simulink model "modified_bouc_wen_sdof"  (R2020a)
settings: Solver=VariableStepAuto  StartTime=0.0  StopTime=10.0  RelTol=1e-3
values from neighbouring files (symbols this model uses):
  A = 301    [modified_bouc_wen_model_parameters.m]
  alpha_a = 140    [modified_bouc_wen_model_parameters.m]
  alpha_b = 695    [modified_bouc_wen_model_parameters.m]
  beta1 = 363    [modified_bouc_wen_model_parameters.m]
  c_0a = 21    [modified_bouc_wen_model_parameters.m]
  c_0b = 3.5    [modified_bouc_wen_model_parameters.m]
  c_1a = 283    [modified_bouc_wen_model_parameters.m]
  c_1b = 2.95    [modified_bouc_wen_model_parameters.m]
  C_s = dr*2*sqrt(m_s*K_s)    [modified_bouc_wen_model_parameters.m]
  eta1 = 190    [modified_bouc_wen_model_parameters.m]
  gamma1 = 363    [modified_bouc_wen_model_parameters.m]
  k0 = 46.9    [modified_bouc_wen_model_parameters.m]
  k1 = 80000    [PID_controller_tov.m]    (also in modified_bouc_wen_model_parameters.m = 5)
  K_s = m_s*((2*pi/T)^2)    (= 155.22913802)    [modified_bouc_wen_model_parameters.m]
  m_s = 98.3    [modified_bouc_wen_model_parameters.m]
  n = 2    [modified_bouc_wen_model_parameters.m]
  x0 = 14.3    [modified_bouc_wen_model_parameters.m]
settings Model: Creator=siddh  LastModifiedBy=siddh

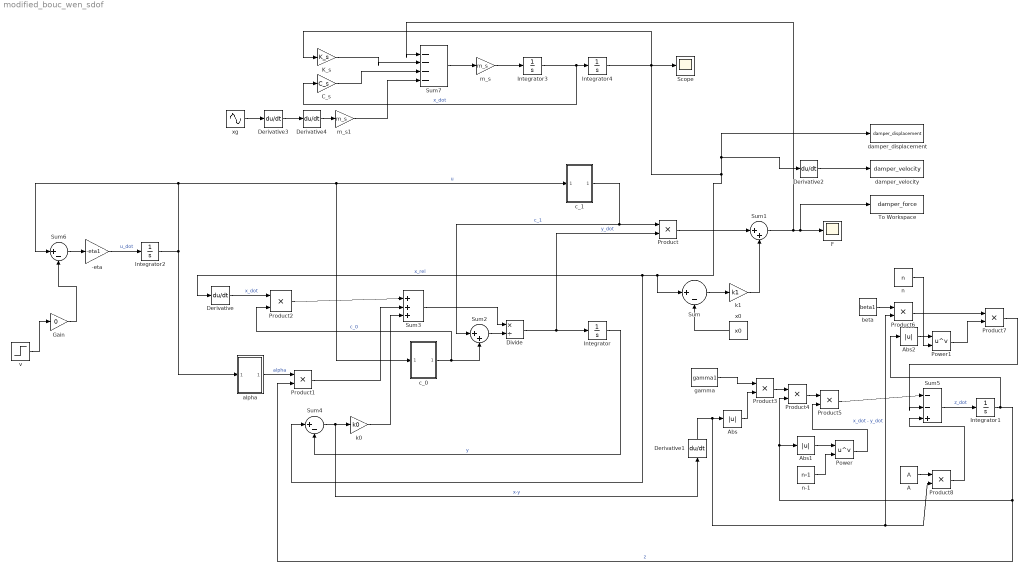
== system modified_bouc_wen_sdof ==
  -eta : Gain  Gain=-eta1
  A : Constant  Value=A
  Abs : Abs
  Abs1 : Abs
  Abs2 : Abs
  C_s : Gain  Gain=C_s
  Derivative{,1..4} (5 alike) : Derivative
  Divide : Product  Inputs=*/
  F : Scope
  Gain : Gain  Gain=0
  Integrator{,1..4} (5 alike) : Integrator
  K_s : Gain  Gain=K_s
  Power : Math  Operator=pow  SaturateOnIntegerOverflow=on
  Power1 : Math  Operator=pow  SaturateOnIntegerOverflow=on
  Product{,1..8} (9 alike) : Product
  Scope : Scope
  Sum : Sum  Inputs=|+-
  Sum1 : Sum  Inputs=|++
  Sum2 : Sum  Inputs=|++
  Sum3 : Sum  Inputs=|+++
  Sum4 : Sum  Inputs=|+-
  Sum5 : Sum  Inputs=|--+
  Sum6 : Sum  Inputs=|+-
  Sum7 : Sum  Inputs=|----
  To Workspace : ToWorkspace  VariableName=damper_force  SampleTime=-1
  alpha : Subsystem
  beta : Constant  Value=beta1
  c_0 : Subsystem
  c_1 : Subsystem
  damper_displacement : ToWorkspace  VariableName=damper_displacement  SampleTime=-1
  damper_velocity : ToWorkspace  VariableName=damper_velocity  SampleTime=-1
  gamma : Constant  Value=gamma1
  k0 : Gain  Gain=k0
  k1 : Gain  Gain=k1
  m_s : Gain  Gain=m_s
  m_s1 : Gain  Gain=m_s
  n : Constant  Value=n
  n-1 : Constant  Value=n-1
  v : Step  SampleTime=0
  x0 : Constant  Value=x0
  xg : Sin  Amplitude=0.75  Frequency=2*pi*4  SampleTime=0
  wires:
  m_s/1 -> Integrator3/1
  Product8/1 -> Sum5/3
  m_s1/1 -> Sum7/4
  Derivative4/1 -> m_s1/1
  A/1 -> Product8/1
  xg/1 -> Derivative3/1
  Product5/1 -> Sum5/1
  Product4/1 -> Product5/1
  C_s/1 -> Sum7/3
  K_s/1 -> Sum7/2
  Sum6/1 -> -eta/1
  n/1 -> Power1/2
  Derivative2/1 -> damper_velocity/1
  v/1 -> Gain/1
  -eta/1 -> Integrator2/1  "u_dot"
  c_1/1(Out1) -> Product/1, Sum2/1  "c_1"
  Product7/1 -> Sum5/2
  Sum/1 -> k1/1
  Integrator4/1 -> Derivative/1, Sum4/1, Sum/1, Derivative2/1, damper_displacement/1, K_s/1, Scope/1  "x_rel"
  Sum7/1 -> m_s/1
  Gain/1 -> Sum6/2
  Derivative3/1 -> Derivative4/1
  x0/1 -> Sum/2
  Abs1/1 -> Power/1
  Integrator/1 -> Sum4/2  "y"
  Sum4/1 -> Derivative1/1, k0/1  "x-y"
  beta/1 -> Product6/1
  Derivative1/1 -> Product8/2, Product6/2, Abs/1  "x_dot - y_dot"
  Product/1 -> Sum1/1
  Product6/1 -> Product7/1
  n-1/1 -> Power/2
  c_0/1(Out1) -> Product2/2, Sum2/2  "c_0"
  gamma/1 -> Product3/1
  Sum5/1 -> Integrator1/1  "z_dot"
  k0/1 -> Sum3/3
  Sum3/1 -> Divide/1
  Product2/1 -> Sum3/1
  alpha/1(Out1) -> Product1/1  "alpha"
  Divide/1 -> Product/2, Integrator/1  "y_dot"
  Abs2/1 -> Power1/1
  Integrator2/1 -> Sum6/1, c_0/1(In1), c_1/1(In1), alpha/1(In1)  "u"
  Abs/1 -> Product3/2
  Integrator1/1 -> Abs2/1, Product4/2, Abs1/1, Product1/2  "z"
  Derivative/1 -> Product2/1  "x_dot"
  Power1/1 -> Product7/2
  Product1/1 -> Sum3/2
  Power/1 -> Product5/2
  k1/1 -> Sum1/2
  Sum2/1 -> Divide/2
  Sum1/1 -> Sum7/1, To Workspace/1, F/1
  Product3/1 -> Product4/1
  Integrator3/1 -> C_s/1, Integrator4/1  "x_dot"

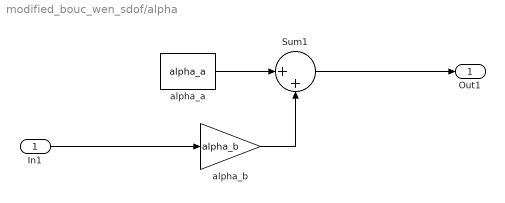
== system modified_bouc_wen_sdof/alpha ==
  In1 : Inport
  Sum1 : Sum  Inputs=|++
  alpha_a : Constant  Value=alpha_a
  alpha_b : Gain  Gain=alpha_b
  Out1 : Outport
  wires:
  In1/1 -> alpha_b/1
  alpha_b/1 -> Sum1/2
  alpha_a/1 -> Sum1/1
  Sum1/1 -> Out1/1

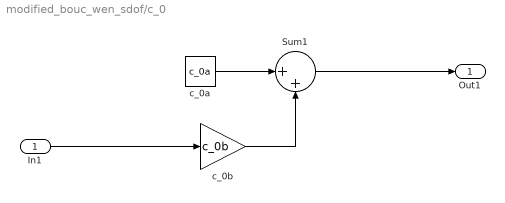
== system modified_bouc_wen_sdof/c_0 ==
  In1 : Inport
  Sum1 : Sum  Inputs=|++
  c_0a : Constant  Value=c_0a
  c_0b : Gain  Gain=c_0b
  Out1 : Outport
  wires:
  Sum1/1 -> Out1/1
  c_0a/1 -> Sum1/1
  c_0b/1 -> Sum1/2
  In1/1 -> c_0b/1

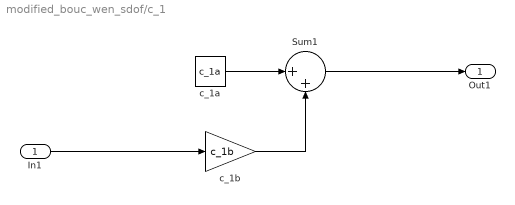
== system modified_bouc_wen_sdof/c_1 ==
  In1 : Inport
  Sum1 : Sum  Inputs=|++
  c_1a : Constant  Value=c_1a
  c_1b : Gain  Gain=c_1b
  Out1 : Outport
  wires:
  In1/1 -> c_1b/1
  c_1b/1 -> Sum1/2
  c_1a/1 -> Sum1/1
  Sum1/1 -> Out1/1
